simulink model "equal_area_criterion_Pm_change"  (R2014a)
settings: Solver=ode23t  StartTime=0.0  StopTime=1  RelTol=1e-3
settings Model: Creator=Divya M  LastModifiedBy=Divya M

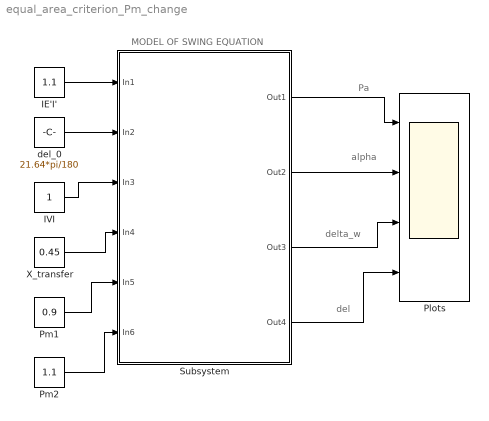
== system equal_area_criterion_Pm_change ==
  note: MODEL OF SWING EQUATION
  note: del
  note: delta_w
  note: alpha
  note: Pa
  IE'I' : Constant  Value=1.1
  IVI : Constant
  Plots : Scope  NumInputPorts=4
      settings: YMin=-0.3~-1000~-10~20  YMax=0.3~1000~10~35
  Pm1 : Constant  Value=0.9
  Pm2 : Constant  Value=1.1
  Subsystem : Subsystem
  X_transfer : Constant  Value=0.45
  del_0 : Constant  Value=21.64*pi/180
  wires:
  IE'I'/1 -> Subsystem/1(In1)
  del_0/1 -> Subsystem/2(In2)
  IVI/1 -> Subsystem/3(In3)
  X_transfer/1 -> Subsystem/4(In4)
  Pm1/1 -> Subsystem/5(In5)
  Pm2/1 -> Subsystem/6(In6)
  Subsystem/1(Out1) -> Plots/1
  Subsystem/2(Out2) -> Plots/2
  Subsystem/3(Out3) -> Plots/3
  Subsystem/4(Out4) -> Plots/4

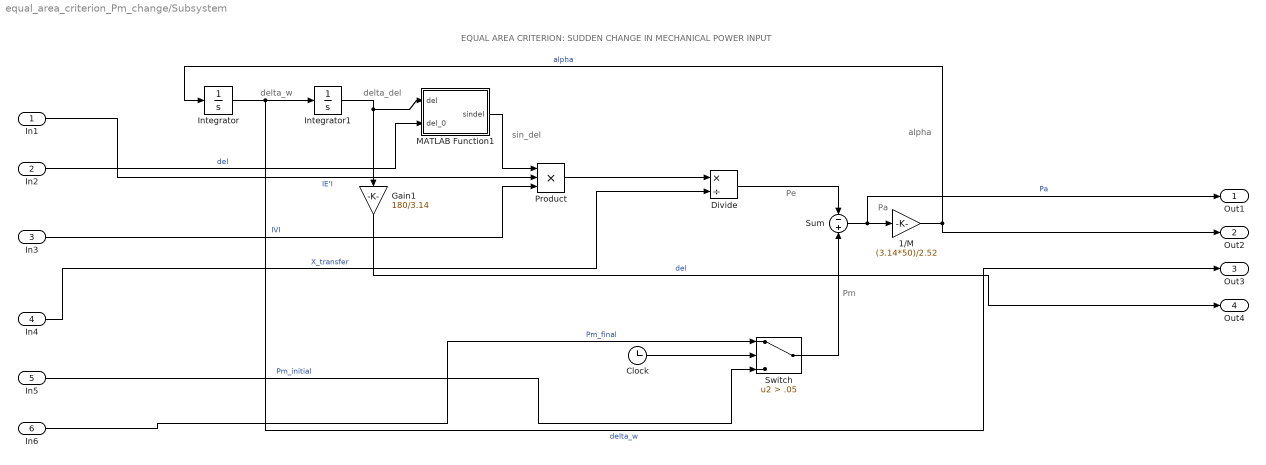
== system equal_area_criterion_Pm_change/Subsystem ==
  note: Pm
  note: alpha
  note: Pa
  note: Pe
  note: sin_del
  note: delta_del
  note: delta_w
  note: EQUAL AREA CRITERION: SUDDEN CHANGE IN MECHANICAL POWER INPUT
  In1 : Inport
  In2 : Inport  Port=2
  In3 : Inport  Port=3
  In4 : Inport  Port=4
  In5 : Inport  Port=5
  In6 : Inport  Port=6
  1/M : Gain  Gain=(3.14*50)/2.52
  Clock : Clock
  Divide : Product  Inputs=*/
  Gain1 : Gain  Gain=180/3.14
  Integrator : Integrator
  Integrator1 : Integrator
  MATLAB Function1 : MATLAB Function  TreatAsAtomicUnit=on
  Product : Product  Inputs=3
  Sum : Sum  Inputs=-+
  Switch : Switch  Criteria=u2 > Threshold  Threshold=.05
  Out1 : Outport
  Out2 : Outport  Port=2
  Out3 : Outport  Port=3
  Out4 : Outport  Port=4
  wires:
  In2/1 -> MATLAB Function1/2(del_0)  "del"
  In1/1 -> Product/2  "IE'I"
  Clock/1 -> Switch/2
  1/M/1 -> Out2/1, Integrator/1  "alpha"
  Divide/1 -> Sum/1
  In5/1 -> Switch/3  "Pm_initial"
  In3/1 -> Product/3  "IVI"
  Switch/1 -> Sum/2
  Integrator/1 -> Out3/1, Integrator1/1  "delta_w"
  Integrator1/1 -> MATLAB Function1/1(del), Gain1/1
  In6/1 -> Switch/1  "Pm_final"
  In4/1 -> Divide/2  "X_transfer"
  Product/1 -> Divide/1
  Gain1/1 -> Out4/1  "del"
  Sum/1 -> Out1/1, 1/M/1  "Pa"
  MATLAB Function1/1(sindel) -> Product/1

== matlab function equal_area_criterion_Pm_change/Subsystem/MATLAB Function1 ==
  data: del input; sindel output; del_0 input
%function y = fcn(u)
function sindel=fcn(del,del_0)
%del0=21.64*pi/180;
del1=del_0+del;
sindel= sin(del1);


%y = u;
